simulink model "ControlLaws_2020a"  (R2020a)
settings: Solver=VariableStepAuto  StartTime=0.0  StopTime=10.0  RelTol=1e-3
undefined symbols (not defined in the file or in its folder): bp, bq, br, cx, cy, cz, g, Jx, Jy, Jz, Kp, Kp2, Kq, Kq2, Kr, Kr2, Kx1, Kx2, Ky1, Ky2, Kz, Kz2, m, z_x, z_y
settings Model: Creator=Asus  LastModifiedBy=alger
settings DebuggingCC: UnconnectedInputMsg=none  UnconnectedOutputMsg=none  UnconnectedLineMsg=none
settings ModelReferenceCC: EnableRefExpFcnMdlSchedulingChecks=off
settings RTWCC: Description=Generic Real-Time Target

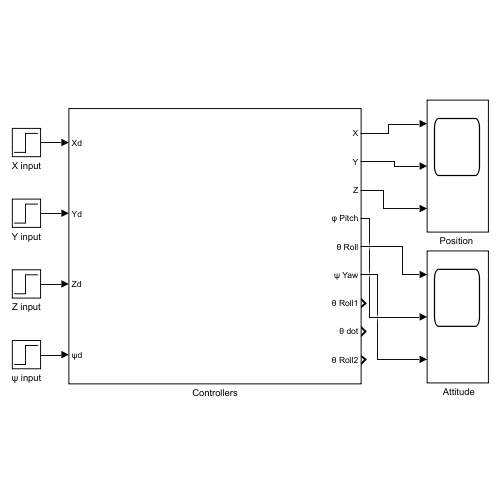
[thumbnail: Simulink's stored preview of the top-level diagram]
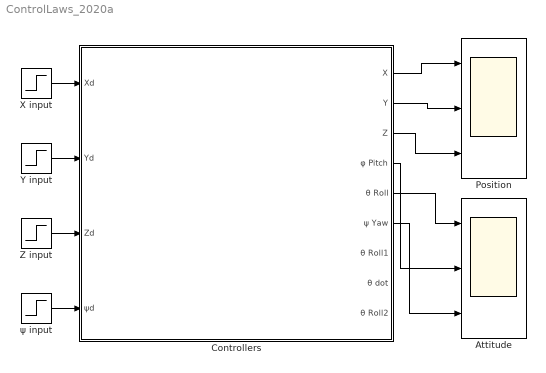
== system ControlLaws_2020a ==
  " Attitude" : Scope  NumInputPorts=3
  Controllers : Subsystem
  "Position " : Scope  NumInputPorts=3
  X input : Step  SampleTime=0
  Y input : Step  After=2  SampleTime=0
  Z input : Step  SampleTime=0
  ψ input : Step  Time=5  After=0.15  SampleTime=0
  wires:
  Controllers/2(Y) -> "Position "/2
  Controllers/3(Z) -> "Position "/3
  Controllers/6(ψ Yaw) -> " Attitude"/3
  ψ input/1 -> Controllers/4(ψd)
  Controllers/1(X) -> "Position "/1
  Y input/1 -> Controllers/2(Yd)
  Z input/1 -> Controllers/3(Zd)
  X input/1 -> Controllers/1(Xd)
  Controllers/4(φ Pitch) -> " Attitude"/2
  Controllers/5(θ Roll) -> " Attitude"/1

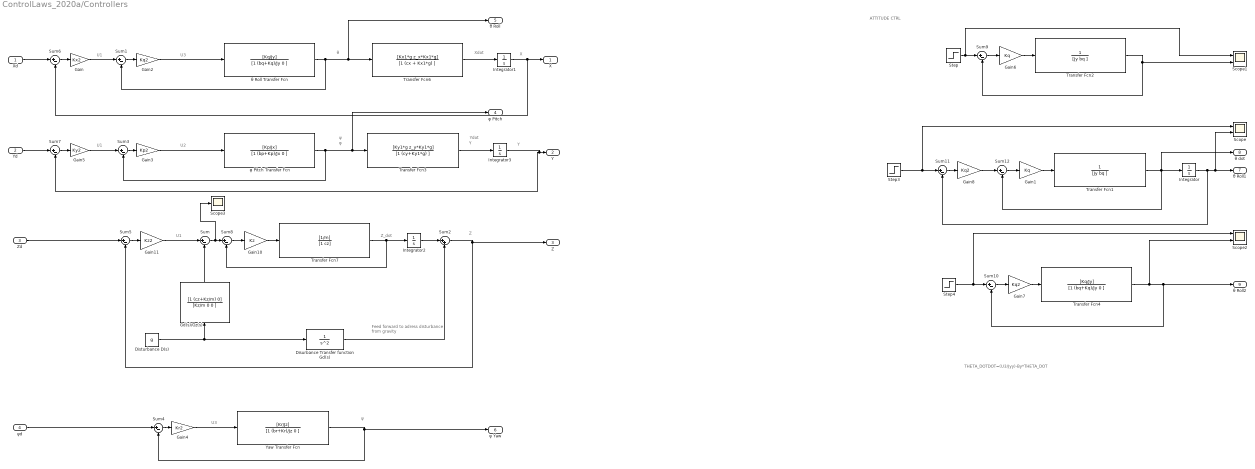
== system ControlLaws_2020a/Controllers ==
  note: THETA_DOTDOT=(U3/Jyy)-By*THETA_DOT
  note: ATTITUDE CTRL
  note: Feed forward to adress disturbance
      | from gravity
  note: φ
  note: U3
  note: U2
  note: U1
  note: U3
  note: Z_dot
  note: ψ
  note: Z
  note: Y
  note: ψ
  note: θ
  note: U1
  note: U1
  note: X
  note: Xdot
  note: Ydot
  note: Y
  Xd : Inport
  Yd : Inport  Port=2
  Zd : Inport  Port=3
  ψd : Inport  Port=4
  Disturbance D(s) : Constant  Value=g
  Disurbance Transfer function Gd(s) : TransferFcn  Denominator=[1 0 0 ]
  Gain : Gain  Gain=Kx2
  Gain1 : Gain  Gain=Kq
  Gain10 : Gain  Gain=Kz
  Gain11 : Gain  Gain=Kz2
  Gain2 : Gain  Gain=Kq2
  Gain3 : Gain  Gain=Kp2
  Gain4 : Gain  Gain=Kr2
  Gain5 : Gain  Gain=Ky2
  Gain6 : Gain  Gain=Kq
  Gain7 : Gain  Gain=Kq2
  Gain8 : Gain  Gain=Kq2
  Gd(s)/Gz(s) : TransferFcn  Numerator=[1 (cz+Kz/m) 0]  Denominator=[Kz/m 0 0 ]
  Integrator{,1..3} (4 alike) : Integrator
  Scope : Scope  NumInputPorts=2
  Scope1 : Scope  NumInputPorts=2
  Scope2 : Scope  NumInputPorts=2
  Scope3 : Scope
  Step : Step  SampleTime=0
  Step3 : Step  SampleTime=0
  Step4 : Step  After=5  SampleTime=0
  Sum{,1,3..12} (12 alike) : Sum  Inputs=|+-
  Sum2 : Sum  Inputs=|++
  Transfer Fcn1 : TransferFcn  Denominator=[Jy bq ]
  Transfer Fcn2 : TransferFcn  Denominator=[Jy bq ]
  Transfer Fcn3 : TransferFcn  Numerator=[Ky1*g z_y*Ky1*g]  Denominator=[1 (cy+Ky1*g) ]
  Transfer Fcn4 : TransferFcn  Numerator=[Kq/Jy]  Denominator=[1 (bq+Kq)/Jy 0 ]
  Transfer Fcn6 : TransferFcn  Numerator=[Kx1*g z_x*Kx1*g]  Denominator=[1 (cx + Kx1*g) ]
  Transfer Fcn7 : TransferFcn  Numerator=[1/m]  Denominator=[1 cz]
  "Yaw Transfer Fcn " : TransferFcn  Numerator=[Kr/Jz]  Denominator=[1 (br+Kr)/Jz 0 ]
  θ Roll Transfer Fcn : TransferFcn  Numerator=[Kq/Jy]  Denominator=[1 (bq+Kq)/Jy 0 ]
  φ Pitch Transfer Fcn : TransferFcn  Numerator=[Kp/Jx]  Denominator=[1 (bp+Kp)/Jx 0 ]
  X : Outport
  Y : Outport  Port=2
  Z : Outport  Port=3
  φ Pitch : Outport  Port=4
  θ Roll : Outport  Port=5
  ψ Yaw : Outport  Port=6
  θ Roll1 : Outport  Port=7
  θ dot : Outport  Port=8
  θ Roll2 : Outport  Port=9
  wires:
  Integrator3/1 -> Sum7/2, Y/1
  Sum7/1 -> Gain5/1
  Sum6/1 -> Gain/1
  Integrator1/1 -> Sum6/2, X/1
  Xd/1 -> Sum6/1
  Yd/1 -> Sum7/1
  θ Roll Transfer Fcn/1 -> Transfer Fcn6/1, θ Roll/1, Sum1/2
  φ Pitch Transfer Fcn/1 -> Transfer Fcn3/1, φ Pitch/1, Sum3/2
  "Yaw Transfer Fcn "/1 -> Sum4/2, ψ Yaw/1
  Gain/1 -> Sum1/1
  Sum1/1 -> Gain2/1
  Gain2/1 -> θ Roll Transfer Fcn/1
  Gain3/1 -> φ Pitch Transfer Fcn/1
  Gain4/1 -> "Yaw Transfer Fcn "/1
  Gain5/1 -> Sum3/1
  Sum3/1 -> Gain3/1
  Sum4/1 -> Gain4/1
  ψd/1 -> Sum4/1
  Gain10/1 -> Transfer Fcn7/1
  Sum8/1 -> Gain10/1
  Transfer Fcn7/1 -> Sum8/2, Integrator2/1
  Integrator2/1 -> Sum2/1
  Sum5/1 -> Gain11/1
  Zd/1 -> Sum5/1
  Gain11/1 -> Sum/1
  Sum/1 -> Scope3/1, Sum8/1
  Disturbance D(s)/1 -> Gd(s)/Gz(s)/1, Disurbance Transfer function Gd(s)/1
  Sum2/1 -> Sum5/2, Z/1
  Disurbance Transfer function Gd(s)/1 -> Sum2/2
  Gd(s)/Gz(s)/1 -> Sum/2
  Transfer Fcn6/1 -> Integrator1/1
  Transfer Fcn3/1 -> Integrator3/1
  Sum9/1 -> Gain6/1
  Transfer Fcn2/1 -> Scope1/2, Sum9/2
  Step/1 -> Sum9/1, Scope1/1
  Gain6/1 -> Transfer Fcn2/1
  Gain1/1 -> Transfer Fcn1/1
  Gain7/1 -> Transfer Fcn4/1
  Gain8/1 -> Sum12/1
  Sum11/1 -> Gain8/1
  Integrator/1 -> θ Roll1/1, Scope/2, Sum11/2
  Step3/1 -> Sum11/1, Scope/1
  Transfer Fcn4/1 -> Sum10/2, θ Roll2/1, Scope2/2
  Sum10/1 -> Gain7/1
  Step4/1 -> Scope2/1, Sum10/1
  Transfer Fcn1/1 -> Integrator/1, θ dot/1, Sum12/2
  Sum12/1 -> Gain1/1
